simulink model "zad1_model_for_linearization"  (Simulink 10.1)
settings: Solver=VariableStepAuto  StartTime=0.0  StopTime=Tsim  RelTol=1e-3
values from neighbouring files (symbols this model uses):
  g = - 9.81    (= -9.81)    [zad1.m]
  h = 0.06    [zad1.m]
  Jh = 0.0021    [zad1.m]
  Jl = 0.0059    [zad1.m]
  Kg = 70    [zad1.m]
  Km = 0.00767    [zad1.m]
  Ks = 1.61    [zad1.m]
  m = 0.4    [zad1.m]
  Rm = 2.6    [zad1.m]
settings Model: Creator=Korisnik  LastModifiedBy=Jakov
settings DataIOCC: SaveFormat=Dataset  ReturnWorkspaceOutputs=on
settings OptimizationCC: LifeSpan=auto
settings DebuggingCC: UnderspecifiedInitializationDetection=Simplified  MergeDetectMultiDrivingBlocksExec=error  UnconnectedInputMsg=none  UnconnectedOutputMsg=none  UnconnectedLineMsg=none  SFUnexpectedBacktrackingDiag=error  SFNoUnconditionalDefaultTransitionDiag=error  SFExecutionAtInitializationDiag=warning  SFMachineParentedDataDiag=error  ArithmeticOperatorsInVariantConditions=error
settings HardwareCC: ProdBitPerPointer=64  ProdBitPerSizeT=64  ProdBitPerPtrDiffT=64  ProdLargestAtomicFloat=Float  ProdIntDivRoundTo=Zero  ProdEndianess=LittleEndian  ProdWordSize=64  ProdHWDeviceType=Intel->x86-64 (Windows64)
settings ModelReferenceCC: PropagateSignalLabelsOutOfModel=on
settings SFSimCC: SimUseLocalCustomCode=on  CustomCodeUndefinedFunction=FilterOut
settings RTWCC: RTWUseLocalCustomCode=on
settings CodeAppCC: StateflowObjectComments=off
settings GRTTargetCC: TargetLangStandard=C99 (ISO)  CombineOutputUpdateFcns=on  GRTInterface=off
settings ConfigComp: CovMetricSettings=dwe  CovSaveCumulativeToWorkspaceVar=off  CovSaveSingleToWorkspaceVar=off  CovExternalEMLEnable=on

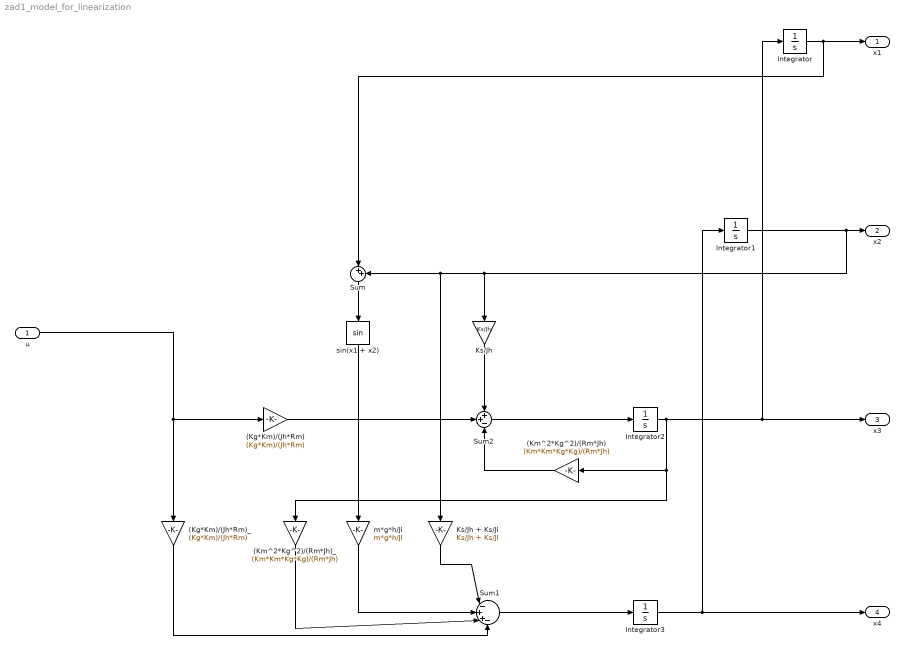
== system zad1_model_for_linearization ==
  u : Inport
  (Kg*Km)/(Jh*Rm) : Gain  Gain=(Kg*Km)/(Jh*Rm)
  (Kg*Km)/(Jh*Rm)_ : Gain  Gain=(Kg*Km)/(Jh*Rm)
  (Km^2*Kg^2)/(Rm*Jh) : Gain  Gain=(Km*Km*Kg*Kg)/(Rm*Jh)
  (Km^2*Kg^2)/(Rm*Jh)_ : Gain  Gain=(Km*Km*Kg*Kg)/(Rm*Jh)
  Integrator{,1..3} (4 alike) : Integrator
  Ks/Jh : Gain  Gain=Ks/Jh
  Ks/Jh + Ks/Jl : Gain  Gain=Ks/Jh + Ks/Jl
  Sum : Sum  Inputs=|++
  Sum1 : Sum  Inputs=|-++-
  Sum2 : Sum  Inputs=++-
  m*g*h/Jl : Gain  Gain=m*g*h/Jl
  sin(x1 + x2) : Trigonometry
  x1 : Outport
  x2 : Outport  Port=2
  x3 : Outport  Port=3
  x4 : Outport  Port=4
  wires:
  Integrator/1 -> Sum/1, x1/1
  Integrator1/1 -> Ks/Jh/1, Ks/Jh + Ks/Jl/1, Sum/2, x2/1
  Integrator2/1 -> x3/1, Integrator/1, (Km^2*Kg^2)/(Rm*Jh)/1, (Km^2*Kg^2)/(Rm*Jh)_/1
  Integrator3/1 -> Integrator1/1, x4/1
  (Km^2*Kg^2)/(Rm*Jh)/1 -> Sum2/3
  (Kg*Km)/(Jh*Rm)/1 -> Sum2/2
  u/1 -> (Kg*Km)/(Jh*Rm)/1, (Kg*Km)/(Jh*Rm)_/1
  Ks/Jh/1 -> Sum2/1
  Sum2/1 -> Integrator2/1
  Sum1/1 -> Integrator3/1
  Ks/Jh + Ks/Jl/1 -> Sum1/1
  m*g*h/Jl/1 -> Sum1/2
  sin(x1 + x2)/1 -> m*g*h/Jl/1
  Sum/1 -> sin(x1 + x2)/1
  (Kg*Km)/(Jh*Rm)_/1 -> Sum1/4
  (Km^2*Kg^2)/(Rm*Jh)_/1 -> Sum1/3
